simulink model "LunarLander_massreduce"  (R2024b)
settings: Solver=ode4  StartTime=0.0  StopTime=100.0  FixedStep=0.01  RelTol=1e-3
settings Model: Creator=max  LastModifiedBy=max
settings DataIOCC: SaveFormat=Array

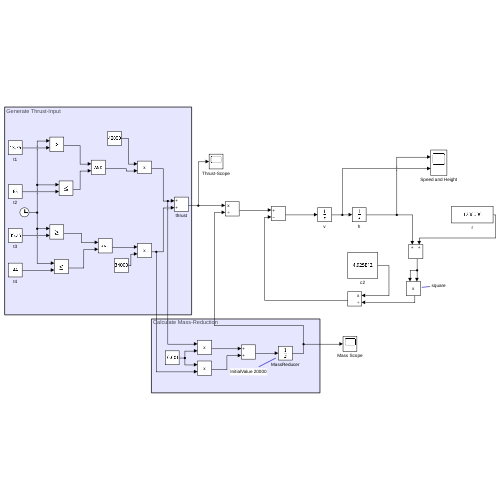
[thumbnail: Simulink's stored preview of the top-level diagram]
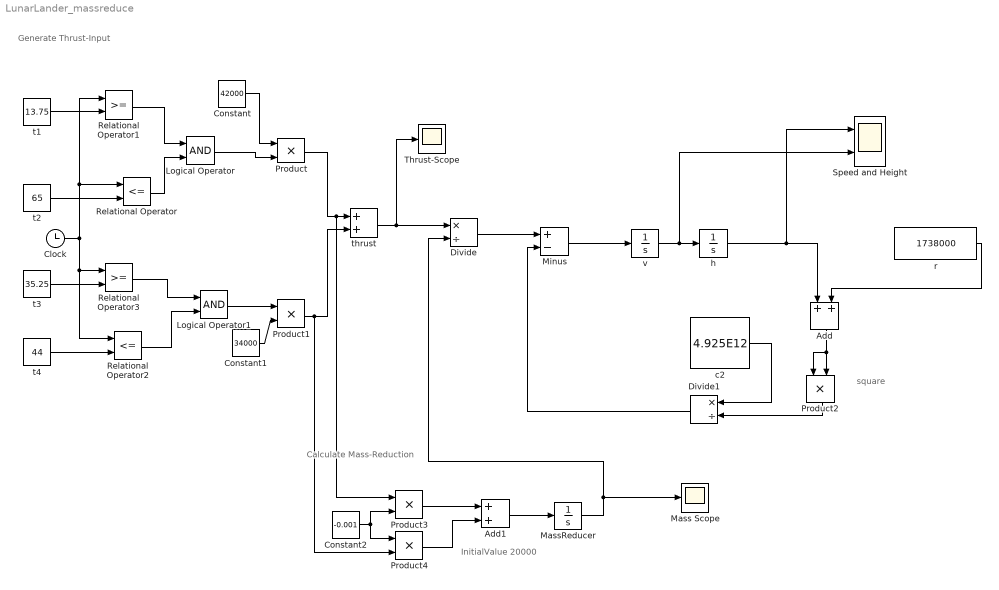
== system LunarLander_massreduce ==
  note: Calculate Mass-Reduction
  note: InitialValue 20000
  note: Generate Thrust-Input
  note: square
  Add : Sum
  Add1 : Sum
  Clock : Clock
  Constant : Constant  Value=42000
  Constant1 : Constant  Value=34000
  Constant2 : Constant  Value=-0.001
  Divide : Product  Inputs=*/
  Divide1 : Product  Inputs=*/
  Logical Operator : Logic  AllPortsSameDT=off  OutDataTypeStr=boolean
  Logical Operator1 : Logic  AllPortsSameDT=off  OutDataTypeStr=boolean
  Mass Scope : Scope
  MassReducer : Integrator  InitialCondition=20000
  Minus : Sum  Inputs=+-
  Product{,1..4} (5 alike) : Product
  Relational Operator : RelationalOperator  Operator=<=  OutDataTypeStr=boolean  RndMeth=Simplest  InputSameDT=off
  Relational Operator1 : RelationalOperator  OutDataTypeStr=boolean  RndMeth=Simplest  InputSameDT=off
  Relational Operator2 : RelationalOperator  Operator=<=  OutDataTypeStr=boolean  RndMeth=Simplest  InputSameDT=off
  Relational Operator3 : RelationalOperator  OutDataTypeStr=boolean  RndMeth=Simplest  InputSameDT=off
  Speed and Height : Scope  NumInputPorts=2
  Thrust-Scope : Scope
  c2 : Constant  Value=4.925E12
  h : Integrator  InitialCondition=1000
  r : Constant  Value=1738000
  t1 : Constant  Value=13.75
  t2 : Constant  Value=65
  t3 : Constant  Value=35.25
  t4 : Constant  Value=44
  thrust : Sum
  v : Integrator  InitialCondition=-10
  wires:
  t1/1 -> Relational Operator1/2
  t2/1 -> Relational Operator/2
  t3/1 -> Relational Operator3/2
  t4/1 -> Relational Operator2/2
  Clock/1 -> Relational Operator2/1, Relational Operator3/1, Relational Operator/1, Relational Operator1/1
  Relational Operator1/1 -> Logical Operator/1
  Relational Operator/1 -> Logical Operator/2
  Relational Operator3/1 -> Logical Operator1/1
  Relational Operator2/1 -> Logical Operator1/2
  Logical Operator/1 -> Product/2
  Logical Operator1/1 -> Product1/1
  Constant/1 -> Product/1
  Constant1/1 -> Product1/2
  Product/1 -> Product3/1, thrust/1
  Product1/1 -> thrust/2, Product4/2
  thrust/1 -> Thrust-Scope/1, Divide/1
  Divide/1 -> Minus/1
  Minus/1 -> v/1
  r/1 -> Add/2
  h/1 -> Speed and Height/1, Add/1
  Add/1 -> Product2/2, Product2/1
  c2/1 -> Divide1/1
  Product2/1 -> Divide1/2
  Divide1/1 -> Minus/2
  v/1 -> Speed and Height/2, h/1
  Add1/1 -> MassReducer/1
  Product3/1 -> Add1/1
  Product4/1 -> Add1/2
  Constant2/1 -> Product4/1, Product3/2
  MassReducer/1 -> Divide/2, Mass Scope/1
